simulink model "slexVariantCondPropToSubsystems"  (R2019b)
settings: Solver=FixedStepAuto  StartTime=0.0  StopTime=10.0  RelTol=1e-3  EnableMultiTasking=on
PreLoadFcn:
  | addpath(fileparts(which(bdroot)));
PostLoadFcn:
  | V = Simulink.Parameter(int32(1));
  | V.StorageClass = 'Define (Custom)';
  | V.CoderInfo.CustomAttributes.HeaderFile='variant_defines.h';
  | 
  | W=copy(V);
libraries: simulink_need_slupdate x3
settings Model: Creator=The MathWorks, Inc.  LastModifiedBy=bhisma
settings DataIOCC: LimitDataPoints=on  SaveFormat=Array  ReturnWorkspaceOutputs=off  OutputSaveName=out1,out2,out3
settings OptimizationCC: LifeSpan=1  EfficientTunableParamExpr=on
settings DebuggingCC: AllowSymbolicDim=off  PregeneratedLibrarySubsystemCodeDiagnostic=none  SFUnexpectedBacktrackingDiag=warning  SFNoUnconditionalDefaultTransitionDiag=warning  SFExecutionAtInitializationDiag=none  ArithmeticOperatorsInVariantConditions=warning
settings HardwareCC: ProdBitPerPointer=32  ProdBitPerSizeT=32  ProdBitPerPtrDiffT=32  ProdLargestAtomicFloat=None  ProdIntDivRoundTo=Undefined  ProdEndianess=Unspecified  ProdWordSize=32  ProdHWDeviceType=32-bit Generic
settings ModelReferenceCC: PropagateSignalLabelsOutOfModel=off
settings SFSimCC: SimUseLocalCustomCode=off  MATLABDynamicMemAlloc=off  CustomCodeUndefinedFunction=UseInterfaceOnly
settings RTWCC: SystemTargetFile=ert.tlc  TemplateMakefile=ert_default_tmf  RTWUseLocalCustomCode=off
settings CodeAppCC: IgnoreCustomStorageClasses=off  CustomSymbolStrModelFcn=$N  StateflowObjectComments=on
settings ERTTargetCC: MultiwordLength=2048  GenerateSampleERTMain=on  MatFileLogging=on  ERTCustomFileTemplate=example_file_process.tlc  ConvertIfToSwitch=off  SuppressUnreachableDefaultCases=off
settings ConfigComp: CovMetricSettings=dw  CovHtmlReporting=on  CovSaveCumulativeToWorkspaceVar=on  CovSaveSingleToWorkspaceVar=on  CovExternalEMLEnable=off

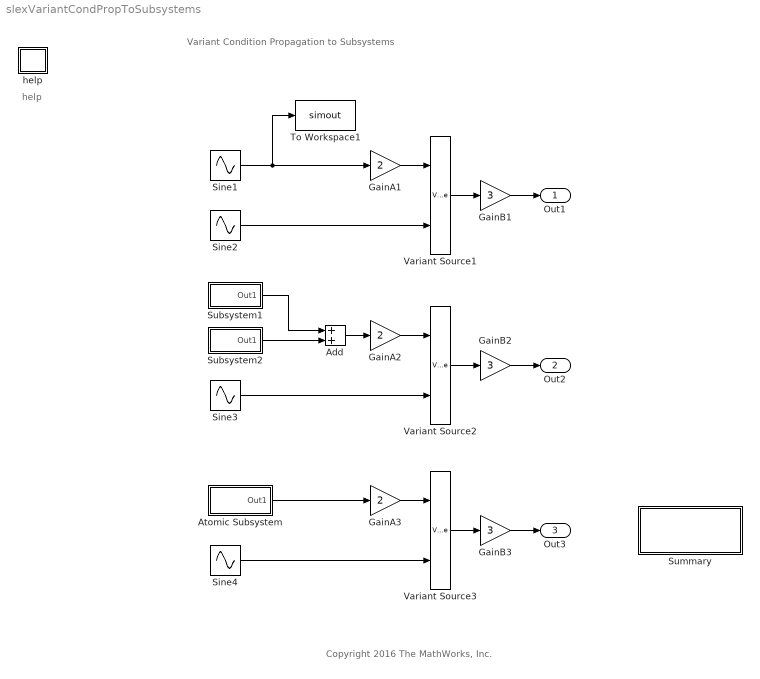
== system slexVariantCondPropToSubsystems ==
  note: Variant Condition Propagation to Subsystems
  note: Copyright 2016 The MathWorks, Inc.
  note: help
  Add : Sum
  Atomic Subsystem : Subsystem  TreatAsAtomicUnit=on
  GainA1 : Gain  Gain=2
  GainA2 : Gain  Gain=2
  GainA3 : Gain  Gain=2
  GainB1 : Gain  Gain=3
  GainB2 : Gain  Gain=3
  GainB3 : Gain  Gain=3
  Sine{1..4} (4 alike) : Sin  SineType=Sample based  SampleTime=0.2
  Subsystem1 : Subsystem
  Subsystem2 : Subsystem
  Summary : Subsystem
  To Workspace1 : ToWorkspace  VariableName=simout  SampleTime=-1
  Variant Source1 : VariantSource
      settings: GeneratePreprocessorConditionals=on
  Variant Source2 : VariantSource
      settings: GeneratePreprocessorConditionals=on
  Variant Source3 : VariantSource
      settings: GeneratePreprocessorConditionals=on
  help : Subsystem
      mask Display: disp('?')
  Out1 : Outport  VectorParamsAs1DForOutWhenUnconnected=off
  Out2 : Outport  Port=2  VectorParamsAs1DForOutWhenUnconnected=off
  Out3 : Outport  Port=3  VectorParamsAs1DForOutWhenUnconnected=off
  wires:
  Sine1/1 -> To Workspace1/1, GainA1/1
  Sine2/1 -> Variant Source1/2
  Variant Source1/1 -> GainB1/1
  GainB1/1 -> Out1/1
  GainA1/1 -> Variant Source1/1
  Sine3/1 -> Variant Source2/2
  Variant Source2/1 -> GainB2/1
  GainB2/1 -> Out2/1
  GainA2/1 -> Variant Source2/1
  Sine4/1 -> Variant Source3/2
  Variant Source3/1 -> GainB3/1
  GainB3/1 -> Out3/1
  GainA3/1 -> Variant Source3/1
  Atomic Subsystem/1(Out1) -> GainA3/1
  Subsystem2/1(Out1) -> Add/2
  Add/1 -> GainA2/1
  Subsystem1/1(Out1) -> Add/1

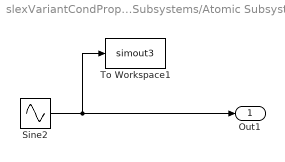
== system slexVariantCondPropToSubsystems/Atomic Subsystem ==
  Sine2 : Sin  SineType=Sample based  SampleTime=0.2
  To Workspace1 : ToWorkspace  VariableName=simout3  SampleTime=-1
  Out1 : Outport  VectorParamsAs1DForOutWhenUnconnected=off
  wires:
  Sine2/1 -> To Workspace1/1, Out1/1

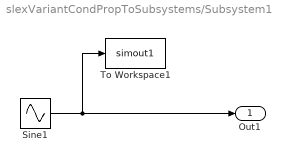
== system slexVariantCondPropToSubsystems/Subsystem1 ==
  Sine1 : Sin  SineType=Sample based  SampleTime=0.2
  To Workspace1 : ToWorkspace  VariableName=simout1  SampleTime=-1
  Out1 : Outport  VectorParamsAs1DForOutWhenUnconnected=off
  wires:
  Sine1/1 -> To Workspace1/1, Out1/1

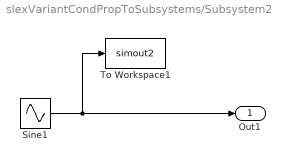
== system slexVariantCondPropToSubsystems/Subsystem2 ==
  Sine1 : Sin  SineType=Sample based  SampleTime=0.2
  To Workspace1 : ToWorkspace  VariableName=simout2  SampleTime=-1
  Out1 : Outport  VectorParamsAs1DForOutWhenUnconnected=off
  wires:
  Sine1/1 -> Out1/1, To Workspace1/1

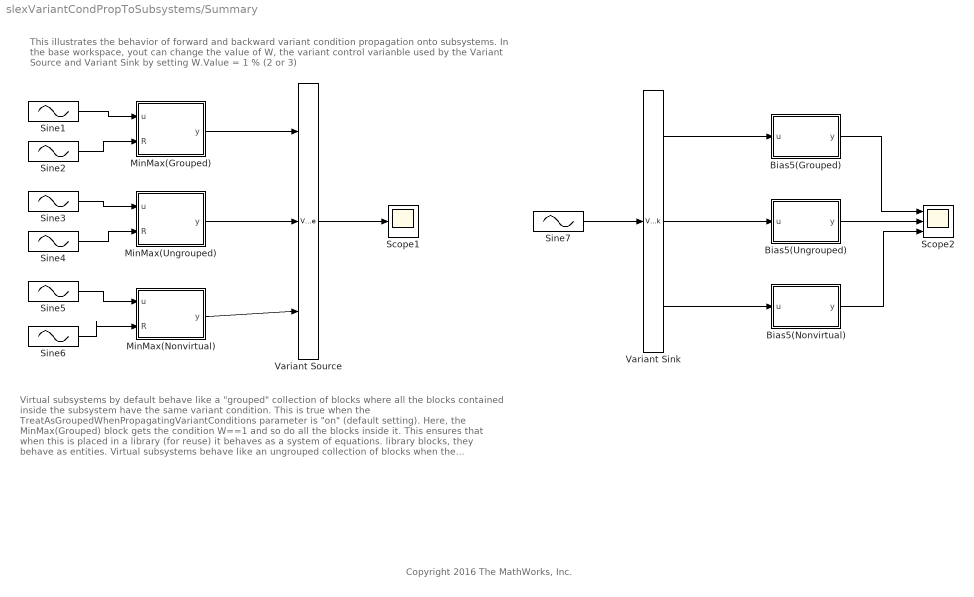
== system slexVariantCondPropToSubsystems/Summary ==
  note: Copyright 2016 The MathWorks, Inc.
  note: This illustrates the behavior of forward and backward variant condition propagation onto subsystems. In the base workspace,
      | yout can change the value of W, the variant control varianble used by the Variant Source and Variant Sink by setting
      | W.Value = 1 % (2 or 3)
  note: Virtual subsystems by default behave like a "grouped" collection of blocks where all the blocks contained inside the subsystem have the same variant condition. This is true when the TreatAsGroupedWhenPropagatingVariantConditions parameter is "on" (default setting). Here, the MinMax(Grouped) block gets the condition W==1 and so do all the blocks inside it. This ensures that when this is placed in a library (for reuse) it behaves as a system of equations. library blocks, they behave as entities.
      | Virtual subsystems behave like an ungrouped collection of blocks when the TreatAsGroupedWhenPropagatingVariantConditions parameter is "off". A dotted line for the MinMax(Ungrouped) block icon indicates this setting. In this example, the behavior of the MinMax(Ungrouped) may not be what one expects in that the block never becomes conditional. Similar for the Bias5(Ungrouped) block in that it does not become conditional.
      | Nonvirtual subsystems always behave like an entity and the contents only execute when the condition assigned to the subsystem is satisfied, i.e. nonvirtual subsystems, Model blocks, and grouped virtual subsystems behave the same.
  Bias5(Grouped) : Subsystem
  "Bias5(Nonvirtual) " : Subsystem  TreatAsAtomicUnit=on
  Bias5(Ungrouped) : Subsystem
  "MinMax(Grouped) " : Subsystem
  MinMax(Nonvirtual) : Subsystem  TreatAsAtomicUnit=on
  "MinMax(Ungrouped) " : Subsystem
  Scope1 : Scope
  Scope2 : Scope  NumInputPorts=3
  Sine{1..7} (7 alike) : Sin  SineType=Sample based  SampleTime=0.2
  Variant Sink : VariantSink
      settings: GeneratePreprocessorConditionals=on
  Variant Source : VariantSource
      settings: GeneratePreprocessorConditionals=on
  wires:
  "MinMax(Ungrouped) "/1(y) -> Variant Source/2
  Variant Source/1 -> Scope1/1
  "MinMax(Grouped) "/1(y) -> Variant Source/1
  Sine1/1 -> "MinMax(Grouped) "/1(u)
  Sine2/1 -> "MinMax(Grouped) "/2(R)
  Sine3/1 -> "MinMax(Ungrouped) "/1(u)
  Sine7/1 -> Variant Sink/1
  Sine4/1 -> "MinMax(Ungrouped) "/2(R)
  Sine5/1 -> MinMax(Nonvirtual)/1(u)
  Sine6/1 -> MinMax(Nonvirtual)/2(R)
  MinMax(Nonvirtual)/1(y) -> Variant Source/3
  Variant Sink/1 -> Bias5(Grouped)/1(u)
  Variant Sink/2 -> Bias5(Ungrouped)/1(u)
  Variant Sink/3 -> "Bias5(Nonvirtual) "/1(u)
  Bias5(Grouped)/1(y) -> Scope2/1
  Bias5(Ungrouped)/1(y) -> Scope2/2
  "Bias5(Nonvirtual) "/1(y) -> Scope2/3

== system slexVariantCondPropToSubsystems/help ==
  note: This illustrates the propagation of variant conditions to subsystems.
      | Variant Source1 has conditions V==1 and V==2 for its input ports. GainA1 is propagated the condition V==1. Similarly, Sine2 is propagated the condition V==2. Notice that Sine1 is unconditional. This is because the To Workspace1 block is unconditional and therefore it's input which is the Sine1 must be unconditional. If we were to comment-out the To Workspace1 block, then Sine1 would be propagated the condition V==1.
      | Subsystem1 and Subsystem2 are virtual subsystems and have identical contents, a Sine Wave connected to a To Workspace and Outport blocks. Subsystem1 has its parameter "Treat as grouped when propagating variant conditions" selected. To access this parameter by right-clicking and selecting the Subsystem1 parameter dialog . This setting specifies that the subsystem represents a well-defined system of equations and therefore the system is propagated the condition V==1. Since Subsystem1 is a system, the condition also applies the blocks within the system.
      | Subsystem2 has its parameter, "Treat as grouped when propagating variant conditions" unselected . This instructs Simulink's variant condition propagation engine to treat the contents of the subsystem as an ungrouped collection of blocks, i.e. it is not meant to represent a system of equations. There is no condition assigned to the Subsystem2 and the conditions are propagated into Subsystem2, resulting in the same conditions as if the subsystem were expanded in place. The dotted lines on the Subsystem2 icon indicate that blocks inside will have ungroped semantics and do not behave like a system.
      | Nonvirtual subsystems (and Model blocks) are always represent a system of equations and thus are handled as a system by variant condition propagation. For example, the conditions propagated to Subsystem1 and the Atomic Subsystem are the same. The Atomic Subsystem contains the same contents as Subsystem1, a Sine Wave connected to a To Workspace and Outport blocks. The system is assigned condition V==1 and therefore its contents only execute when V==1.
      | The propagations of conditions to subsystems is the same when pbackwards propagation as shown to the left, or forward propagation as shown in the Summary subsystem.

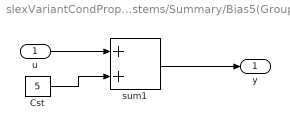
== system slexVariantCondPropToSubsystems/Summary/Bias5(Grouped) ==
  u : Inport
  Cst : Constant  Value=5
  sum1 : Sum  SaturateOnIntegerOverflow=on  InputSameDT=on  OutDataTypeStr=Inherit: Same as first input
  y : Outport  VectorParamsAs1DForOutWhenUnconnected=off
  wires:
  u/1 -> sum1/1
  Cst/1 -> sum1/2
  sum1/1 -> y/1

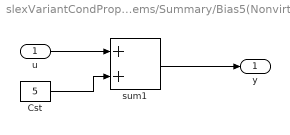
== system slexVariantCondPropToSubsystems/Summary/Bias5(Nonvirtual)  ==
  u : Inport
  Cst : Constant  Value=5
  sum1 : Sum  SaturateOnIntegerOverflow=on  InputSameDT=on  OutDataTypeStr=Inherit: Same as first input
  y : Outport  VectorParamsAs1DForOutWhenUnconnected=off
  wires:
  u/1 -> sum1/1
  Cst/1 -> sum1/2
  sum1/1 -> y/1

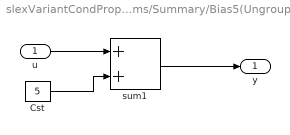
== system slexVariantCondPropToSubsystems/Summary/Bias5(Ungrouped) ==
  u : Inport
  Cst : Constant  Value=5
  sum1 : Sum  SaturateOnIntegerOverflow=on  InputSameDT=on  OutDataTypeStr=Inherit: Same as first input
  y : Outport  VectorParamsAs1DForOutWhenUnconnected=off
  wires:
  u/1 -> sum1/1
  Cst/1 -> sum1/2
  sum1/1 -> y/1

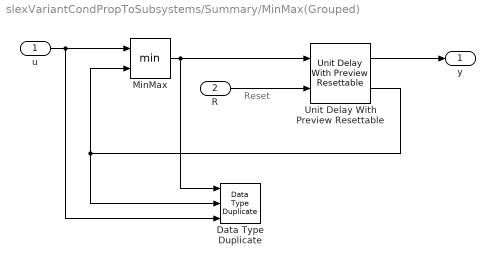
== system slexVariantCondPropToSubsystems/Summary/MinMax(Grouped)  ==
  note: Reset
  u : Inport
  R : Inport  Port=2
  Data Type Duplicate : DataTypeDuplicate  DisableCoverage=on  NumInputPorts=3
  MinMax : MinMax  DisableCoverage=on  Inputs=2  OutDataTypeStr=Inherit: Inherit via back propagation  ZeroCross=off
      settings: LockScale=on
  Unit Delay With Preview Resettable : simulink_need_slupdate/Unit Delay With Preview Resettable  vinit=0.0  tsamp=-1
      settings: SourceProductName=Simulink  SourceProductBaseCode=SL
  y : Outport  VectorParamsAs1DForOutWhenUnconnected=off
  wires:
  Unit Delay With Preview Resettable/1 -> y/1
  MinMax/1 -> Unit Delay With Preview Resettable/1, Data Type Duplicate/1
  Unit Delay With Preview Resettable/2 -> MinMax/2, Data Type Duplicate/2
  u/1 -> MinMax/1, Data Type Duplicate/3
  R/1 -> Unit Delay With Preview Resettable/2

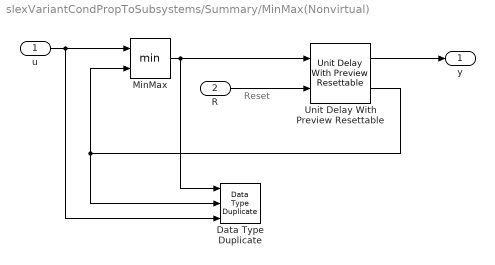
== system slexVariantCondPropToSubsystems/Summary/MinMax(Nonvirtual) ==
  note: Reset
  u : Inport
  R : Inport  Port=2
  Data Type Duplicate : DataTypeDuplicate  DisableCoverage=on  NumInputPorts=3
  MinMax : MinMax  DisableCoverage=on  Inputs=2  OutDataTypeStr=Inherit: Inherit via back propagation  ZeroCross=off
      settings: LockScale=on
  Unit Delay With Preview Resettable : simulink_need_slupdate/Unit Delay With Preview Resettable  vinit=1  tsamp=-1
      settings: SourceProductName=Simulink  SourceProductBaseCode=SL
  y : Outport  VectorParamsAs1DForOutWhenUnconnected=off
  wires:
  Unit Delay With Preview Resettable/1 -> y/1
  MinMax/1 -> Unit Delay With Preview Resettable/1, Data Type Duplicate/1
  Unit Delay With Preview Resettable/2 -> MinMax/2, Data Type Duplicate/2
  u/1 -> MinMax/1, Data Type Duplicate/3
  R/1 -> Unit Delay With Preview Resettable/2

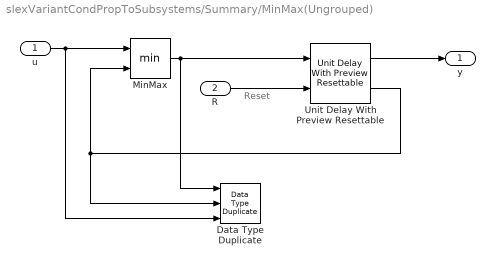
== system slexVariantCondPropToSubsystems/Summary/MinMax(Ungrouped)  ==
  note: Reset
  u : Inport
  R : Inport  Port=2
  Data Type Duplicate : DataTypeDuplicate  DisableCoverage=on  NumInputPorts=3
  MinMax : MinMax  DisableCoverage=on  Inputs=2  OutDataTypeStr=Inherit: Inherit via back propagation  ZeroCross=off
      settings: LockScale=on
  Unit Delay With Preview Resettable : simulink_need_slupdate/Unit Delay With Preview Resettable  vinit=1  tsamp=-1
      settings: SourceProductName=Simulink  SourceProductBaseCode=SL
  y : Outport  VectorParamsAs1DForOutWhenUnconnected=off
  wires:
  Unit Delay With Preview Resettable/1 -> y/1
  MinMax/1 -> Unit Delay With Preview Resettable/1, Data Type Duplicate/1
  Unit Delay With Preview Resettable/2 -> MinMax/2, Data Type Duplicate/2
  u/1 -> MinMax/1, Data Type Duplicate/3
  R/1 -> Unit Delay With Preview Resettable/2
